simulink model "mondmission"  (Simulink 8.5)
settings: Solver=ode45  StartTime=0.0  StopTime=500000  MaxStep=100  RelTol=1e-3
settings Model: Creator=aas547  LastModifiedBy=Abdre
settings DataIOCC: SignalLoggingSaveFormat=Dataset
settings OptimizationCC: ExpressionDepthLimit=128
settings DebuggingCC: SolverPrmCheckMsg=warning  FcnCallInpInsideContextMsg=EnableAllAsError  StateNameClashWarn=none
settings GRTTargetCC: CombineOutputUpdateFcns=on  GRTInterface=off

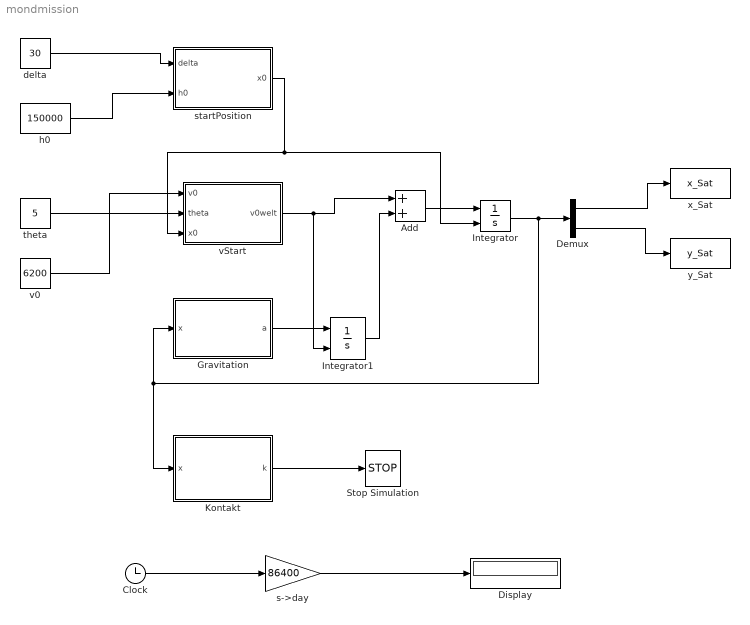
== system mondmission ==
  Add : Sum
  Clock : Clock
  Demux : Demux  Outputs=2
  Display : Display
  Gravitation : MATLAB Function  TreatAsAtomicUnit=on
  Integrator : Integrator  InitialConditionSource=external
  Integrator1 : Integrator  InitialConditionSource=external
  Kontakt : MATLAB Function  TreatAsAtomicUnit=on
  Stop Simulation : Stop
  delta : Constant  Value=30
  h0 : Constant  Value=150000
  s->day : Gain  Gain=86400
  startPosition : MATLAB Function  TreatAsAtomicUnit=on
  theta : Constant  Value=5
  v0 : Constant  Value=6200
  "vStart " : MATLAB Function  TreatAsAtomicUnit=on
  x_Sat : ToWorkspace  VariableName=x_Sat  SampleTime=-1
  y_Sat : ToWorkspace  VariableName=y_Sat  SampleTime=-1
  wires:
  Clock/1 -> s->day/1
  s->day/1 -> Display/1
  delta/1 -> startPosition/1(delta)
  h0/1 -> startPosition/2(h0)
  theta/1 -> "vStart "/2(theta)
  startPosition/1(x0) -> Integrator/2, "vStart "/3(x0)
  Integrator/1 -> Kontakt/1(x), Gravitation/1(x), Demux/1
  "vStart "/1(v0welt) -> Integrator1/2, Add/1
  Gravitation/1(a) -> Integrator1/1
  Integrator1/1 -> Add/2
  Add/1 -> Integrator/1
  Demux/1 -> x_Sat/1
  Demux/2 -> y_Sat/1
  Kontakt/1(k) -> Stop Simulation/1
  v0/1 -> "vStart "/1(v0)

== matlab function vStart  ==
  data: v0 input double; v0welt output double; theta input double; x0 input double
function v0welt = vStart(v0,theta,x0)
thetaBog = theta * pi/180;
n = x0/norm(x0);
t = [n(2);-n(1)];
vn = sin(thetaBog) * v0;
vt = cos(thetaBog) * v0;
v0welt = vn * n + vt * t;

== matlab function startPosition ==
  data: delta input double; x0 output double; h0 input double
function x0 = Startposition(delta,h0)
deltaBog = delta * pi/180;
rE = 6378137;
x0 = [cos(deltaBog)*(h0+rE);sin(deltaBog)*(h0+rE)];

== matlab function Gravitation ==
  data: x input double; a output double
function a = Gravitation(x)
mE = 5.9736*10^24;
mM = 7.3480*10^22;
G = 66.743*10^-12;
eSE = - x/norm(x);
SM = - x + [0;380000000];
eSM = SM / norm(SM);
aE = (G * mE * eSE) / (norm(x)^2);
aM = (G * mM * eSM) / (norm(SM)^2);
a = aE + aM;

== matlab function Kontakt ==
  data: x input double; k output double
function k = Kontakt(x)
rE = 6378137;
if (norm(x) > rE)
    k = 0;
else
    k = 1;
end
